simulink library "EngineSystemSubmodel"  (R2014b)
settings: Solver=ode45  StartTime=0.0  StopTime=10.0  FixedStep=1e-4  RelTol=1e-3
values from neighbouring files (symbols this model uses):
  D_turb_wheel = TC.TC_map.turb.D_wheel    [init_MVM.m]
  delta = 2    [Init8RTFLEX68D.m]    (also in Untitled2.m = fcn(p); fcn.m = zeros(size(p)))
  eta_turb_max = TC.TC_map.turb.eff_max    [init_MVM.m]
  flow_coeff_turb = [-1.585326540339;-4.823836967181;1.5853156139822]    [Init8RTFLEX68D.m]    (also in init_MVM.m = TC.TC_map.turb.flow_fit_coeff)
  fs = 0.0683    [Init8RTFLEX68D.m]    (also in NOxProcessGUI.m = varargin{2}; initHybrid.m; initMV.m; init_MVM.m = 0.0682925799315)
  genset = generators(1)    [runTempCyl4S.m]
  J_tc = TC.SAE_map_comp.inertia    [init_MVM.m]
  kai = 1.7    [Init8RTFLEX68D.m]
  Kb = 1*ones(engines,1)    [initHybrid.m]    (also in initMV.m; init_MVM.m = 1; init_ele.m = 1)
  Kd = 20*ones(engines,1)    [initHybrid.m]    (also in initMV.m; init_MVM.m = 10; init_ele.m = 20)
  Ki = 20*ones(engines,1)    [initHybrid.m]    (also in initMV.m; init_MVM.m = 10; init_ele.m = 20)
  Kp = 20*ones(engines,1)    [initHybrid.m]    (also in initMV.m; init_MVM.m = 10; init_ele.m = 20)
  Load_amp = x(4) + xRef(i)    [GetErrGensetResp.m]    (also in runsimulation.m = 0.55; runsimulationRecovery.m = InitialLoad(jj) + LoadStep(ii))
  Load_bias = x(4)    [GetErrGensetResp.m]    (also in runsimulation.m = 0.15; runsimulationRecovery.m = InitialLoad(jj))
  Load_index = 1    [GetErrGensetResp.m]    (also in runsimulation.m; runsimulationRecovery.m)
  N = x*noMol    [NOxProcessGUI.m]    (also in initHybrid.m = .1*ones(engines,1); initMV.m = .1*ones(engines,1); init_ele.m = 0.1)
  omegat0 = RPM_TC_initial/30*pi    [init_MVM.m]
  Start_time = 50    [GetErrGensetResp.m]    (also in runsimulation.m; runsimulationRecovery.m)
  T_load = 1    [GetErrGensetResp.m]    (also in runsimulation.m; runsimulationRecovery.m)
  T_ref_turb = TC.TC_map.turb.T_ref    [init_MVM.m]
  u0 = 0.2    [init_MVM.m]
  Uc_opt = TC.TC_map.turb.Uc_opt    [init_MVM.m]
  uMax = 1.5*ones(engines,1)    [initHybrid.m]    (also in initMV.m; init_MVM.m = 1.1; init_ele.m = 1.1)
  uMin = 0*ones(engines,1)    [initHybrid.m]    (also in initMV.m; init_MVM.m = 0.1; init_ele.m = 0.1)
undefined symbols (not defined in the file or in its folder): CAIPO, control, CV, cyl, eng, engSCont, omega0, rhoG0, Td, Ti, turbo, u_max, volDisp, vSCont, vSDes
undefined symbols (not defined in the file): comp_eff_map, comp_flow_map, n288_rep, npr, nsp, pr_rep, vComp
libraries: EngineSystemSubmodel x167, simulink x2
(part 4 of 5)

== system EngineSystemSubmodel/Components/TurbochargerFullModel ==
  pTFuComp : Inport
  pTFdComp : Inport  Port=2
  pTFuTurb : Inport  Port=3
  pTFdTurb : Inport  Port=4
  CompressorFullMap : EngineSystemSubmodel/Flow Restriction/CompressorFullMap  comp=turbo.comp
  Friction : Subsystem
  Gain : Gain  Gain=1/turbo.jTC
  Integrator : Integrator  InitialCondition=turbo.jTC*turbo.omegaT0
  Sum : Sum  Inputs=--+
  TurbineFullMap : EngineSystemSubmodel/Flow Restriction/TurbineFullMap  turb=turbo.turb
  dmEmbuComp : Outport
  dmEmbdComp : Outport  Port=2
  effComp : Outport  Port=3
  effComp1 : Outport  Port=4
  dmEmbuTurb : Outport  Port=5
  dmEmbdTurb : Outport  Port=6
  effTurb : Outport  Port=7
  TdTurb : Outport  Port=8
  wires:
  Integrator/1 -> Gain/1
  TurbineFullMap/3 -> Sum/3  "tqTurb"
  Sum/1 -> Integrator/1
  TurbineFullMap/4 -> effTurb/1  "etaTurb"
  Gain/1 -> TurbineFullMap/3, CompressorFullMap/3, Friction/1(In1)  "omegaTC"
  pTFdTurb/1 -> TurbineFullMap/2
  CompressorFullMap/3 -> Sum/2  "tqComp"
  TurbineFullMap/2 -> dmEmbdTurb/1
  pTFuComp/1 -> CompressorFullMap/1
  CompressorFullMap/1 -> dmEmbuComp/1
  pTFuTurb/1 -> TurbineFullMap/1
  CompressorFullMap/2 -> dmEmbdComp/1
  CompressorFullMap/4 -> effComp/1  "etaComp"
  pTFdComp/1 -> CompressorFullMap/2
  TurbineFullMap/1 -> dmEmbuTurb/1
  Friction/1(Out1) -> Sum/1  "tqFricTC"
  TurbineFullMap/5 -> TdTurb/1  "TAComp"
  CompressorFullMap/5 -> effComp1/1

== system EngineSystemSubmodel/Components/TurbochargerMV ==
  pTF_c_u : Inport
  pTF_c_d : Inport  Port=2
  pTF_t_u : Inport  Port=3
  pTF_t_d : Inport  Port=4
  Compressor : EngineSystemSubmodel/Flow Restriction/Compressor  comp=turbo.comp
  Gain : Gain  Gain=1/J_tc
  Integrator : Integrator  InitialCondition=omegat0*J_tc
  Sum : Sum  Inputs=-|+
  TurbineMV : EngineSystemSubmodel/Flow Restriction/TurbineMV  fs=fs  flow_coeff_turb=flow_coeff_turb  D_turb_wheel=D_turb_wheel  Uc_opt=Uc_opt  eta_turb_max=eta_turb_max
  dmEmb_c_u : Outport
  dmEmb_c_d : Outport  Port=2
  dmEmb_t_u : Outport  Port=3
  dmEmb_t_d : Outport  Port=4
  T_t_d_calc : Outport  Port=5
  eta_c : Outport  Port=6
  eta_t : Outport  Port=7
  wires:
  TurbineMV/5 -> eta_t/1
  TurbineMV/3 -> Sum/2  "Tqt"
  TurbineMV/1 -> dmEmb_t_u/1
  Compressor/1 -> dmEmb_c_u/1
  Gain/1 -> Compressor/3, TurbineMV/3  "omegat"
  Compressor/2 -> dmEmb_c_d/1
  Integrator/1 -> Gain/1
  Sum/1 -> Integrator/1
  Compressor/3 -> Sum/1  "Tqc"
  TurbineMV/2 -> dmEmb_t_d/1
  TurbineMV/4 -> T_t_d_calc/1
  pTF_c_d/1 -> Compressor/2
  pTF_c_u/1 -> Compressor/1
  pTF_t_u/1 -> TurbineMV/1
  pTF_t_d/1 -> TurbineMV/2
  Compressor/4 -> eta_c/1

== system EngineSystemSubmodel/Components/WasteGate ==
  pTF_u : Inport
  pTF_d : Inport  Port=2
  pTFScav : Inport  Port=3
  dmEmbExh : Inport  Port=4
  Demux : Demux  Outputs=3
  Demux1 : Demux  Outputs=3
  Demux2 : Demux  Outputs=3
  IdealNozzle : EngineSystemSubmodel/Flow Restriction/IdealNozzle
  S-Function : S-Function  FunctionName=lowPassFilterBW4  Parameters=BW,y0  EnableBusSupport=off  mask{BW=eng.control.WG.LPBWdmExhBypass, y0=0}
      mask prompts: BW "Bandwidth [Hz]"; y0 "Initial output"
  S-Function1 : S-Function  FunctionName=lowPassFilterBW4  Parameters=BW,y0  EnableBusSupport=off  mask{BW=eng.control.WG.LPBWdmExh, y0=0}
      mask prompts: BW "Bandwidth [Hz]"; y0 "Initial output"
  Terminator{,1..5} (6 alike) : Terminator
  wasteGateControl : Subsystem  mask{Kp=eng.control.WG.Kp, Ti=eng.control.WG.Ti, K_b=eng.control.WG.Kb, max=eng.control.WG.uMax, min=eng.control.WG.uMin, bypassRatio=eng.control.WG.Ratio, upper=eng.control.WG.upperOpenSPWG, lower=eng.control.WG.lowerCloseSPWG}
      mask prompts: Kp "Proportional gain"; Ti "Integral time constant"; K_b "Back calculation gain for anti-windup"; max "Maximum allowable valve opening"; min "Maximum allowable valve opening"; bypassRatio "Bypass ratio"; upper "Upper bound for opening waste gate"; lower "Lower bound for closing waste gate"
      mask TypeOptions Kp: Gain/Kp | Gain2/Kp
      mask TypeOptions Ti: Gain1/Ti
      mask TypeOptions K_b: Gain3/K_b
      mask TypeOptions max: Saturation/max
      mask TypeOptions min: Saturation/min
      mask TypeOptions bypassRatio: Constant1/bypassRatio
      mask TypeOptions upper: S-Function/upper
      mask TypeOptions lower: S-Function/lower
  dmEmb_u : Outport
  dmEmb_d : Outport  Port=2
  wires:
  Demux2/3 -> Terminator5/1
  Demux2/2 -> Terminator4/1
  Demux2/1 -> S-Function1/1
  dmEmbExh/1 -> Demux2/1
  Demux1/3 -> Terminator3/1
  Demux1/2 -> Terminator2/1
  Demux1/1 -> S-Function/1
  IdealNozzle/2 -> Demux1/1, dmEmb_d/1
  Demux/3 -> Terminator1/1
  Demux/2 -> Terminator/1
  Demux/1 -> wasteGateControl/3(pScav)
  S-Function/1 -> wasteGateControl/1(dmExhBypass)
  pTFScav/1 -> Demux/1
  S-Function1/1 -> wasteGateControl/2(dmExhTotal)
  pTF_d/1 -> IdealNozzle/3
  pTF_u/1 -> IdealNozzle/2
  wasteGateControl/1(wasteGateOpen) -> IdealNozzle/1, wasteGateControl/4(u saturated)
  IdealNozzle/1 -> dmEmb_u/1

== system EngineSystemSubmodel/Control System/ECSParamId ==
  Tq : Inport
  omegaE : Inport  Port=2
  RPMRef : Inport  Port=3
  dmf : Inport  Port=4
  pMax : Inport  Port=5
  pCyl : Inport  Port=6
  vCyl : Inport  Port=7
  exhVVOpen : Inport  Port=8
  dQCyl : Inport  Port=9
  BSFCRef : Inport  Port=10
  dQCylREf : Inport  Port=11
  Constant : Constant  Value=1e-6
  Constant1 : Constant  Value=exhVVStart  mask{exhVVStart=eng.control.EVO}
      mask prompts: exhVVStart "EVO timing (0.96~1.2)"
  Constant4 : Constant  Value=deltaPCombRef  mask{deltaPCombRef=control.inj.deltaPCombRef}
      mask prompts: deltaPCombRef "Reference pressure rise due to combustion"
  EVCControl : Subsystem  mask{Kp=control.EVC.Kp, Ti=control.EVC.Ti, max=control.EVC.uMax, min=control.EVC.uMin}
      mask prompts: Kp "Proportional gain"; Ti "Integral time constant"; max "Maximum allowable output"; min "Minimum allowable output"
  Gain : Gain  Gain=30/pi/eng.RPMMax
  Gain1 : Gain  Gain=1e-5
  Gain2 : Gain  Gain=3.6e9
  Gain3 : Gain  Gain=1e-5
  Gain4 : Gain  Gain=1/eng.RPMMax
  Gain5 : Gain  Gain=1/eng.nCyl
  InjectionControl : Subsystem  mask{Kp=control.inj.Kp, Ti=control.inj.Ti, max=control.inj.uMax, min=control.inj.uMin}
      mask prompts: Kp "Proportional gain"; Ti "Integral time constant"; max "Maximum allowable output"; min "Minimum allowable output"
  PIDControlAntiWinding : EngineSystemSubmodel/Control System/PIDControlAntiWinding  Kp=control.gov.Kp  Td=control.gov.Td  N=control.gov.N  Ti=control.gov.Ti  uMax=control.gov.uMax  uMin=control.gov.uMin  u0=control.gov.u0  Kb=control.gov.Kb
  Product : Product  Inputs=*/
  Product1 : Product
  Sum : Sum  Inputs=|++
  Sum1 : Sum  Inputs=|+-
  Sum2 : Sum  Inputs=|-+
  dQCylLPFilterBW1 : S-Function  FunctionName=lowPassFilterBW4  Parameters=BW,y0  EnableBusSupport=off  mask{BW=eng.control.HRejId.LPBWQCyl, y0=0}
      mask prompts: BW "Bandwidth [Hz]"; y0 "Initial output"
  dmfLPFilterBW4 : S-Function  FunctionName=lowPassFilterBW4  Parameters=BW,y0  EnableBusSupport=off  mask{BW=eng.control.pMax.LPBWdmf, y0=eng.BSFC0*(eng.engLoad0*eng.Pe)/3.6e9}
      mask prompts: BW "Bandwidth [Hz]"; y0 "Initial output"
  engSpeedLPFilterBW1 : S-Function  FunctionName=lowPassFilterBW4  Parameters=BW,y0  EnableBusSupport=off  mask{BW=100, y0=0}
      mask prompts: BW "Bandwidth [Hz]"; y0 "Initial output"
  engSpeedLPFilterBW4 : S-Function  FunctionName=lowPassFilterBW4  Parameters=BW,y0  EnableBusSupport=off  mask{BW=eng.control.gov.LPBW, y0=eng.omegaE0}
      mask prompts: BW "Bandwidth [Hz]"; y0 "Initial output"
  maxPCylMaxControl : Subsystem  mask{Kp=control.pMax.Kp, Ti=control.pMax.Ti, max=control.pMax.uMax, min=control.pMax.uMin}
      mask prompts: Kp "Proportional gain"; Ti "Integral time constant"; max "Maximum allowable output"; min "Minimum allowable output"
  pCompCalc : EngineSystemSubmodel/EngineOperatingParameterCalculation/pCompCalc  vComp=eng.cyl(1).dim.vComp
  powLPFilterBW4 : S-Function  FunctionName=lowPassFilterBW4  Parameters=BW,y0  EnableBusSupport=off  mask{BW=eng.control.pMax.LPBWPow, y0=eng.engLoad0*eng.Pe}
      mask prompts: BW "Bandwidth [Hz]"; y0 "Initial output"
  tempWallControl : Subsystem  mask{Kp=control.HRejId.Kp, Ti=control.HRejId.Ti, swTWCont=control.HRejId.sw}
      mask prompts: Kp "Proportional gain"; Ti "Integral time constant"; swTWCont "Switch ON/OFF for TWall identification"
  uGov : Outport
  phiInj : Outport  Port=2
  cAStartNom : Outport  Port=3
  dCALiftUp : Outport  Port=4
  TWall : Outport  Port=5
  wires:
  Gain5/1 -> tempWallControl/2(dQCylRef)  "dQCyl1Ref"
  Gain4/1 -> PIDControlAntiWinding/2  "engSpeedRefPU"
  Gain/1 -> PIDControlAntiWinding/1  "engSpeedPU"
  Gain1/1 -> EVCControl/1(pComp)  "pCompBar"
  engSpeedLPFilterBW1/1 -> Gain1/1, Sum1/2  "pComp"
  BSFCRef/1 -> maxPCylMaxControl/2(BSFCRef)  "BSFCREf"
  omegaE/1 -> Product1/1, engSpeedLPFilterBW4/1
  engSpeedLPFilterBW4/1 -> Gain/1  "omegaELP"
  RPMRef/1 -> Gain4/1
  PIDControlAntiWinding/1 -> PIDControlAntiWinding/3, uGov/1  "uGov"
  Product1/1 -> powLPFilterBW4/1  "powInst"
  Constant1/1 -> cAStartNom/1  "CAStartNom"
  powLPFilterBW4/1 -> Sum/2  "powLP"
  dmf/1 -> dmfLPFilterBW4/1
  Sum/1 -> Product/2
  Product/1 -> Gain2/1
  Gain2/1 -> maxPCylMaxControl/1(BSFCMeas)  "BSFC"
  pCyl/1 -> pCompCalc/1
  vCyl/1 -> pCompCalc/2
  tempWallControl/1(TWall) -> pCompCalc/3, TWall/1  "tempWall"
  pMax/1 -> Sum1/1
  Sum1/1 -> Gain3/1  "deltaPComb"
  Gain3/1 -> InjectionControl/1(deltaPComb), Sum2/1
  maxPCylMaxControl/1(pMaxRef) -> Sum2/2  "pMaxRef"
  Sum2/1 -> EVCControl/2(pCompRef)  "pCompRef"
  Constant4/1 -> InjectionControl/2(deltaPCombRef)
  Tq/1 -> Product1/2
  dmfLPFilterBW4/1 -> Product/1  "dmfLP"
  Constant/1 -> Sum/1
  exhVVOpen/1 -> pCompCalc/4
  pCompCalc/1 -> engSpeedLPFilterBW1/1
  InjectionControl/1(phiInjRef) -> phiInj/1  "phiInj"
  EVCControl/1(EVCRef) -> dCALiftUp/1  "EVC"
  dQCyl/1 -> dQCylLPFilterBW1/1
  dQCylLPFilterBW1/1 -> tempWallControl/1(dQCyl)  "dQCyl1"
  dQCylREf/1 -> Gain5/1

== system EngineSystemSubmodel/Control System/ECSTrans ==
  Tq : Inport
  omegaE : Inport  Port=2
  RPMRef : Inport  Port=3
  dmf : Inport  Port=4
  dme : Inport  Port=5
  Constant : Constant  Value=1e-6
  Constant1 : Constant  Value=exhVVStart  mask{exhVVStart=control.EVO}
      mask prompts: exhVVStart "EVO timing (0.96~1.2)"
  Gain : Gain  Gain=30/pi/eng.RPMMax
  Gain1 : Gain  Gain=1/eng.Pe
  Gain2 : Gain  Gain=3.6e9
  Gain3 : Gain  Gain=3.6e6
  Gain4 : Gain  Gain=1/eng.RPMMax
  PIDControlAntiWinding : EngineSystemSubmodel/Control System/PIDControlAntiWinding  Kp=control.gov.Kp  Td=control.gov.Td  N=control.gov.N  Ti=control.gov.Ti  uMax=control.gov.uMax  uMin=control.gov.uMin  u0=control.gov.u0  Kb=control.gov.Kb
  Product : Product  Inputs=*/
  Product1 : Product
  Product2 : Product  Inputs=*/
  S-Function : S-Function  FunctionName=interpolateDescend  Parameters=xREf,yRef  EnableBusSupport=off  mask{xREf=eng.control.inj.phiInjxRef, yRef=eng.control.inj.phiInjyRef}
      mask prompts: xREf "x Reference array to interpolate"; yRef "y Reference array to interpolate"
  S-Function1 : S-Function  FunctionName=interpolateDescend  Parameters=xREf,yRef  EnableBusSupport=off  mask{xREf=eng.control.EVC.EVCxRef, yRef=eng.control.EVC.EVCyRef}
      mask prompts: xREf "x Reference array to interpolate"; yRef "y Reference array to interpolate"
  S-Function2 : S-Function  FunctionName=lowPassFilterBW4  Parameters=BW,y0  EnableBusSupport=off  mask{BW=eng.control.dmfLP.BW, y0=eng.BSFC0*(eng.engLoad0*eng.Pe)/3.6e9}
      mask prompts: BW "Bandwidth [Hz]"; y0 "Initial output"
  S-Function3 : S-Function  FunctionName=lowPassFilterBW4  Parameters=BW,y0  EnableBusSupport=off  mask{BW=eng.control.powLP.BW, y0=eng.control.powLP.pow0}
      mask prompts: BW "Bandwidth [Hz]"; y0 "Initial output"
  S-Function4 : S-Function  FunctionName=lowPassFilterBW4  Parameters=BW,y0  EnableBusSupport=off  mask{BW=eng.control.gov.LPBW, y0=eng.omegaE0}
      mask prompts: BW "Bandwidth [Hz]"; y0 "Initial output"
  S-Function5 : S-Function  FunctionName=lowPassFilterBW4  Parameters=BW,y0  EnableBusSupport=off  mask{BW=eng.control.dmeLP.BW, y0=eng.control.dmeLP.dme0}
      mask prompts: BW "Bandwidth [Hz]"; y0 "Initial output"
  Sum : Sum  Inputs=|++
  Terminator1 : Terminator
  Terminator2 : Terminator
  uGov : Outport
  phiInj : Outport  Port=2
  cAStartNom : Outport  Port=3
  dCALiftUp : Outport  Port=4
  wires:
  Gain3/1 -> Terminator1/1  "BSEF"
  Product2/1 -> Gain3/1
  S-Function5/1 -> Product2/1  "dmeLP"
  dme/1 -> S-Function5/1
  omegaE/1 -> Product1/1, S-Function4/1
  S-Function4/1 -> Gain/1  "omegaELP"
  Gain/1 -> PIDControlAntiWinding/1  "engSpeedPU"
  RPMRef/1 -> Gain4/1
  PIDControlAntiWinding/1 -> PIDControlAntiWinding/3, uGov/1  "uGov"
  Product1/1 -> S-Function3/1  "powInst"
  Constant1/1 -> cAStartNom/1
  S-Function3/1 -> Product2/2, Sum/2, Gain1/1  "powLP"
  Gain1/1 -> S-Function1/1, S-Function/1  "PL"
  dmf/1 -> S-Function2/1
  Sum/1 -> Product/2
  Product/1 -> Gain2/1
  Gain2/1 -> Terminator2/1  "BSFC"
  Gain4/1 -> PIDControlAntiWinding/2  "engSpeedRefPU"
  Tq/1 -> Product1/2
  S-Function2/1 -> Product/1  "dmfLP"
  Constant/1 -> Sum/1
  S-Function/1 -> phiInj/1
  S-Function1/1 -> dCALiftUp/1

== system EngineSystemSubmodel/Control System/ECSTrans1 ==
  Tq : Inport
  omegaE : Inport  Port=2
  RPMRef : Inport  Port=3
  dmf : Inport  Port=4
  dme : Inport  Port=5
  vS : Inport  Port=6
  vSRef : Inport  Port=7
  Constant : Constant  Value=1e-6
  Constant1 : Constant  Value=exhVVStart  mask{exhVVStart=eng.control.EVO}
      mask prompts: exhVVStart "EVO timing (0.96~1.2)"
  Gain : Gain  Gain=30/pi/eng.RPMMax
  Gain1 : Gain  Gain=1/eng.Pe
  Gain11 : Gain  Gain=vSCont
  Gain12 : Gain  Gain=engSCont
  Gain2 : Gain  Gain=3.6e9
  Gain3 : Gain  Gain=3.6e6
  Gain4 : Gain  Gain=1/eng.RPMMax
  Gain8 : Gain  Gain=1/vSDes
  Integrator : Integrator
  PIDControlAntiWinding : EngineSystemSubmodel/Control System/PIDControlAntiWinding  Kp=control.gov.Kp  Td=control.gov.Td  N=control.gov.N  Ti=control.gov.Ti  uMax=control.gov.uMax  uMin=control.gov.uMin  u0=control.gov.u0  Kb=control.gov.Kb
  PIDControlAntiWinding1 : EngineSystemSubmodel/Control System/PIDControlAntiWinding  Kp=control.speed.Kp  Td=control.speed.Td  N=control.speed.N  Ti=control.speed.Ti  uMax=control.speed.uMax  uMin=control.speed.uMin  u0=control.speed.u0  Kb=control.speed.Kb
  Product : Product  Inputs=*/
  Product1 : Product
  Product2 : Product  Inputs=*/
  S-Function : S-Function  FunctionName=interpolateDescend  Parameters=xREf,yRef  EnableBusSupport=off  mask{xREf=eng.control.inj.phiInjxRef, yRef=eng.control.inj.phiInjyRef}
      mask prompts: xREf "x Reference array to interpolate"; yRef "y Reference array to interpolate"
  S-Function1 : S-Function  FunctionName=interpolateDescend  Parameters=xREf,yRef  EnableBusSupport=off  mask{xREf=eng.control.EVC.EVCxRef, yRef=eng.control.EVC.EVCyRef}
      mask prompts: xREf "x Reference array to interpolate"; yRef "y Reference array to interpolate"
  S-Function2 : S-Function  FunctionName=lowPassFilterBW4  Parameters=BW,y0  EnableBusSupport=off  mask{BW=eng.control.dmfLP.BW, y0=eng.BSFC0*(eng.engLoad0*eng.Pe)/3.6e9}
      mask prompts: BW "Bandwidth [Hz]"; y0 "Initial output"
  S-Function3 : S-Function  FunctionName=lowPassFilterBW4  Parameters=BW,y0  EnableBusSupport=off  mask{BW=eng.control.powLP.BW, y0=eng.control.powLP.pow0}
      mask prompts: BW "Bandwidth [Hz]"; y0 "Initial output"
  S-Function4 : S-Function  FunctionName=lowPassFilterBW4  Parameters=BW,y0  EnableBusSupport=off  mask{BW=eng.control.gov.LPBW, y0=eng.omegaE0}
      mask prompts: BW "Bandwidth [Hz]"; y0 "Initial output"
  S-Function5 : S-Function  FunctionName=lowPassFilterBW4  Parameters=BW,y0  EnableBusSupport=off  mask{BW=eng.control.dmeLP.BW, y0=eng.control.dmeLP.dme0}
      mask prompts: BW "Bandwidth [Hz]"; y0 "Initial output"
  S-Function6 : EngineSystemSubmodel/Control System/ECSTrans1/S-Function4  BW=eng.control.speed.LPBW  y0=vS0
  Sum : Sum  Inputs=|++
  Sum2 : Sum  Inputs=|++
  Terminator : Terminator
  Terminator1 : Terminator
  Terminator2 : Terminator
  uGov : Outport
  phiInj : Outport  Port=2
  cAStartNom : Outport  Port=3
  dCALiftUp : Outport  Port=4
  wires:
  S-Function1/1 -> dCALiftUp/1
  S-Function/1 -> phiInj/1
  Constant/1 -> Sum/1
  S-Function2/1 -> Product/1  "dmfLP"
  Tq/1 -> Product1/2
  Gain4/1 -> PIDControlAntiWinding/2  "engSpeedRefPU"
  Gain2/1 -> Terminator2/1  "BSFC"
  Product/1 -> Gain2/1
  Sum/1 -> Product/2
  dmf/1 -> S-Function2/1
  Gain1/1 -> S-Function/1, S-Function1/1  "PL"
  S-Function3/1 -> Gain1/1, Sum/2, Product2/2  "powLP"
  Constant1/1 -> cAStartNom/1
  Product1/1 -> Integrator/1, S-Function3/1  "powInst"
  RPMRef/1 -> Gain4/1
  Gain/1 -> PIDControlAntiWinding/1  "engSpeedPU"
  S-Function4/1 -> Gain/1  "omegaELP"
  omegaE/1 -> S-Function4/1, Product1/1
  dme/1 -> S-Function5/1
  S-Function5/1 -> Product2/1  "dmeLP"
  Product2/1 -> Gain3/1
  Gain3/1 -> Terminator1/1  "BSEF"
  Integrator/1 -> Terminator/1  "workShaft"
  Sum2/1 -> uGov/1
  Gain12/1 -> Sum2/2
  Gain11/1 -> Sum2/1
  PIDControlAntiWinding1/1 -> PIDControlAntiWinding1/3, Gain11/1
  Gain8/1 -> PIDControlAntiWinding1/1
  S-Function6/1 -> Gain8/1
  vS/1 -> S-Function6/1
  vSRef/1 -> PIDControlAntiWinding1/2
  PIDControlAntiWinding/1 -> PIDControlAntiWinding/3, Gain12/1

== system EngineSystemSubmodel/Control System/ECSTransSmokeLim ==
  Tq : Inport
  omegaE : Inport  Port=2
  RPMRef : Inport  Port=3
  dmf : Inport  Port=4
  dme : Inport  Port=5
  vS : Inport  Port=6
  vSRef : Inport  Port=7
  pTFVAR : Inport  Port=8
  volEff : Inport  Port=9
  Bus Selector : BusSelector  OutputSignals=p,T
  Compare To Constant : simulink/Logic and Bit Operations/Compare To Constant  relop=<=  const=(eng.RPMMax/30*pi)*0.1  OutDataTypeStr=boolean
  Constant : Constant  Value=1e-6
  Constant1 : Constant  Value=exhVVStart  mask{exhVVStart=eng.control.EVO}
      mask prompts: exhVVStart "EVO timing (0.96~1.2)"
  Gain : Gain  Gain=30/pi/eng.RPMMax
  Gain1 : Gain  Gain=1/eng.Pe
  Gain11 : Gain  Gain=vSCont
  Gain12 : Gain  Gain=engSCont
  Gain2 : Gain  Gain=3.6e9
  Gain3 : Gain  Gain=3.6e6
  Gain4 : Gain  Gain=1/eng.RPMMax
  Gain5 : Gain  Gain=vSCont
  Gain6 : Gain  Gain=engSCont
  Gain8 : Gain  Gain=1/vSDes
  Integrator : Integrator
  PIDControlAntiWinding : EngineSystemSubmodel/Control System/PIDControlAntiWinding  Kp=control.gov.Kp  Td=control.gov.Td  N=control.gov.N  Ti=control.gov.Ti  uMax=control.gov.uMax  uMin=control.gov.uMin  u0=control.gov.u0  Kb=control.gov.Kb
  PIDControlAntiWinding1 : EngineSystemSubmodel/Control System/PIDControlAntiWinding  Kp=control.speed.Kp  Td=control.speed.Td  N=control.speed.N  Ti=control.speed.Ti  uMax=control.speed.uMax  uMin=control.speed.uMin  u0=control.speed.u0  Kb=control.speed.Kb
  Product : Product  Inputs=*/
  Product1 : Product
  Product2 : Product  Inputs=*/
  S-Function : S-Function  FunctionName=interpolateDescend  Parameters=xREf,yRef  EnableBusSupport=off  mask{xREf=eng.control.inj.phiInjxRef, yRef=eng.control.inj.phiInjyRef}
      mask prompts: xREf "x Reference array to interpolate"; yRef "y Reference array to interpolate"
  S-Function1 : S-Function  FunctionName=interpolateDescend  Parameters=xREf,yRef  EnableBusSupport=off  mask{xREf=eng.control.EVC.EVCxRef, yRef=eng.control.EVC.EVCyRef}
      mask prompts: xREf "x Reference array to interpolate"; yRef "y Reference array to interpolate"
  S-Function2 : S-Function  FunctionName=lowPassFilterBW4  Parameters=BW,y0  EnableBusSupport=off  mask{BW=eng.control.dmfLP.BW, y0=eng.BSFC0*(eng.engLoad0*eng.Pe)/3.6e9}
      mask prompts: BW "Bandwidth [Hz]"; y0 "Initial output"
  S-Function3 : S-Function  FunctionName=lowPassFilterBW4  Parameters=BW,y0  EnableBusSupport=off  mask{BW=eng.control.powLP.BW, y0=eng.control.powLP.pow0}
      mask prompts: BW "Bandwidth [Hz]"; y0 "Initial output"
  S-Function4 : S-Function  FunctionName=lowPassFilterBW4  Parameters=BW,y0  EnableBusSupport=off  mask{BW=eng.control.gov.LPBW, y0=eng.omegaE0}
      mask prompts: BW "Bandwidth [Hz]"; y0 "Initial output"
  S-Function5 : S-Function  FunctionName=lowPassFilterBW4  Parameters=BW,y0  EnableBusSupport=off  mask{BW=eng.control.dmeLP.BW, y0=eng.control.dmeLP.dme0}
      mask prompts: BW "Bandwidth [Hz]"; y0 "Initial output"
  S-Function6 : EngineSystemSubmodel/Control System/ECSTrans1/S-Function4  BW=eng.control.speed.LPBW  y0=vS0
  Smoke Limiter : EngineSystemSubmodel/Control System/Smoke Limiter
  Stop Simulation : Stop
  Sum : Sum  Inputs=|++
  Sum2 : Sum  Inputs=|++
  Terminator{,1..3} (4 alike) : Terminator
  uGov : Outport
  phiInj : Outport  Port=2
  cAStartNom : Outport  Port=3
  dCALiftUp : Outport  Port=4
  wires:
  Compare To Constant/1 -> Stop Simulation/1
  PIDControlAntiWinding/1 -> Gain12/1
  vSRef/1 -> PIDControlAntiWinding1/2
  vS/1 -> S-Function6/1
  S-Function6/1 -> Gain8/1
  Gain8/1 -> PIDControlAntiWinding1/1
  PIDControlAntiWinding1/1 -> Gain11/1
  Gain11/1 -> Sum2/1
  Gain12/1 -> Sum2/2
  Sum2/1 -> Smoke Limiter/1
  Integrator/1 -> Terminator/1  "workShaft"
  Gain3/1 -> Terminator1/1  "BSEF"
  Product2/1 -> Gain3/1
  S-Function5/1 -> Product2/1  "dmeLP"
  dme/1 -> S-Function5/1
  omegaE/1 -> Product1/1, S-Function4/1, Compare To Constant/1
  S-Function4/1 -> Gain/1  "omegaELP"
  Gain/1 -> PIDControlAntiWinding/1  "engSpeedPU"
  RPMRef/1 -> Gain4/1
  Product1/1 -> S-Function3/1, Integrator/1  "powInst"
  Constant1/1 -> cAStartNom/1
  S-Function3/1 -> Product2/2, Sum/2, Gain1/1  "powLP"
  Gain1/1 -> S-Function1/1, S-Function/1  "PL"
  dmf/1 -> S-Function2/1
  Sum/1 -> Product/2
  Product/1 -> Gain2/1
  Gain2/1 -> Terminator2/1  "BSFC"
  Gain4/1 -> PIDControlAntiWinding/2  "engSpeedRefPU"
  Tq/1 -> Product1/2
  S-Function2/1 -> Product/1  "dmfLP"
  Constant/1 -> Sum/1
  S-Function/1 -> phiInj/1
  S-Function1/1 -> dCALiftUp/1
  Smoke Limiter/1 -> Gain5/1, Gain6/1, uGov/1  "uGov"
  volEff/1 -> Smoke Limiter/4
  pTFVAR/1 -> Bus Selector/1
  Bus Selector/2 -> Smoke Limiter/3  "<T>"
  Bus Selector/1 -> Smoke Limiter/2  "<p>"
  Gain5/1 -> PIDControlAntiWinding1/3
  Gain6/1 -> PIDControlAntiWinding/3
  Smoke Limiter/2 -> Terminator3/1  "uMax"

== system EngineSystemSubmodel/Control System/Governor ==
  u saturated : Inport
  omega_pu : Inport  Port=2
  "wNL, pu" : Inport  Port=3
  "pe, pu" : Inport  Port=4
  Constant : Constant
  Gain : Gain  Gain=genset.governor.droop
  PID controller : Subsystem
  Product : Product  RndMeth=Zero
  Sum : Sum  Inputs=|+-
  Sum1 : Sum  Inputs=|+-
  u : Outport
  wires:
  omega_pu/1 -> PID controller/2(omega_pu), Sum/2
  "pe, pu"/1 -> Gain/1
  u saturated/1 -> PID controller/3(u saturated)
  Sum1/1 -> Product/2
  Constant/1 -> Sum1/1
  "wNL, pu"/1 -> Product/1
  Product/1 -> Sum/1
  Sum/1 -> PID controller/1(e)
  Gain/1 -> Sum1/2
  PID controller/1(u) -> u/1  "u"

== system EngineSystemSubmodel/Control System/Governor_SpeedControl ==
  u saturated : Inport
  omega_pu : Inport  Port=2
  omega_pu_ref : Inport  Port=3
  PID controller : Subsystem  mask{Kp=Kp, Kd=Kd, N=N, Ki=Ki, Kb=Kb, omega0=omega0, u_max=u_max, u_min=u_min, u0=u0}
      mask prompts: Kp "Proportional gain"; Kd "Differtial gain"; N "Dirty derivative gain"; Ki "Integral gain"; Kb "Back-calculation gain"; omega0 "Initial speed"; u_max "Maximum output"; u_min "Minimum output"; u0 "Initial output"
  Sum : Sum  Inputs=|+-
  u : Outport
  wires:
  omega_pu/1 -> PID controller/2(omega_pu), Sum/2
  u saturated/1 -> PID controller/3(u saturated)
  omega_pu_ref/1 -> Sum/1
  Sum/1 -> PID controller/1(e)  "error"
  PID controller/1(u) -> u/1

== system EngineSystemSubmodel/Control System/PIDControlAntiWinding ==
  MV : Inport
  SP : Inport  Port=2
  uSat : Inport  Port=3
  S-Function : S-Function  FunctionName=SpeedController  Parameters=Kp,Td,N,Ti,Kb,uMax,uMin,u0  EnableBusSupport=off
  output : Outport
  wires:
  S-Function/1 -> output/1
  uSat/1 -> S-Function/3
  SP/1 -> S-Function/2
  MV/1 -> S-Function/1

== system EngineSystemSubmodel/Control System/Smoke Limiter ==
  u_gov : Inport
  p_air_manifold : Inport  Port=2
  T_air_manifold : Inport  Port=3
  vol_eff : Inport  Port=4
  Disp. Vol : Gain  Gain=eng.cyl(1).dim.vDisp
  Divide : Product  Inputs=/*
  Gain : Gain  Gain=eng.fs
  Gain1 : Gain  Gain=eng.control.smokeLim.FMax
  Gain2 : Gain  Gain=1/eng.cyl(1).comb.mqfCycMax
  LPFilterBW1 : EngineSystemSubmodel/Control System/LPFilterBW4  BW=eng.control.smokeLim.LPBW  y0=eng.scavRec.p0
  LPFilterBW4 : EngineSystemSubmodel/Control System/LPFilterBW4  BW=eng.control.smokeLim.LPBW  y0=eng.scavRec.T0
  LP_T0_2 : Subsystem
  MinMax : MinMax  Inputs=2
  Product : Product
  R_air : Gain  Gain=287
  u : Outport
  u_max : Outport  Port=2
  wires:
  LP_T0_2/1(Out1) -> Product/2
  LPFilterBW1/1 -> Divide/2
  LPFilterBW4/1 -> R_air/1
  Divide/1 -> Disp. Vol/1  "rho_air"
  p_air_manifold/1 -> LPFilterBW1/1
  R_air/1 -> Divide/1
  T_air_manifold/1 -> LPFilterBW4/1
  Disp. Vol/1 -> Product/1  "m_air_ideal"
  MinMax/1 -> u/1  "u"
  vol_eff/1 -> LP_T0_2/1(In1)  "eta_vol"
  Product/1 -> Gain/1  "m_a_cyl"
  u_gov/1 -> MinMax/1
  Gain/1 -> Gain1/1  "m_f_st"
  Gain1/1 -> Gain2/1  "m_f_max"
  Gain2/1 -> u_max/1, MinMax/2  "u_max"

== system EngineSystemSubmodel/Control System/Smoke Limiter MV ==
  u_gov : Inport
  p_air_manifold : Inport  Port=2
  T_air_manifold : Inport  Port=3
  vol_eff : Inport  Port=4
  Disp. Vol : Gain  Gain=Vd
  Divide : Product  Inputs=/*
  Gain : Gain  Gain=fs
  Gain1 : Gain  Gain=F_max
  Gain2 : Gain  Gain=1/m_f_cyc_max
  LP_T0_01 : Subsystem
  LP_T0_1 : Subsystem
  LP_T0_2 : Subsystem
  MinMax : MinMax  Inputs=2
  Product : Product
  R_air : Gain  Gain=287
  u : Outport
  u_max : Outport  Port=2
  wires:
  LP_T0_2/1(Out1) -> Product/2
  LP_T0_1/1(Out1) -> Divide/2
  LP_T0_01/1(Out1) -> R_air/1
  Divide/1 -> Disp. Vol/1  "rho_air"
  p_air_manifold/1 -> LP_T0_1/1(In1)
  R_air/1 -> Divide/1
  T_air_manifold/1 -> LP_T0_01/1(In1)
  Disp. Vol/1 -> Product/1  "m_air_ideal"
  MinMax/1 -> u/1  "u"
  vol_eff/1 -> LP_T0_2/1(In1)  "eta_vol"
  Product/1 -> Gain/1  "m_a_cyl"
  u_gov/1 -> MinMax/1
  Gain/1 -> Gain1/1  "m_f_st"
  Gain1/1 -> Gain2/1  "m_f_max"
  Gain2/1 -> u_max/1, MinMax/2  "u_max"

== system EngineSystemSubmodel/Control System/SpeedController ==
  MV : Inport
  SP : Inport  Port=2
  Demux : Demux  Outputs=[1 ]
  Mux : Mux  Inputs=[1 1 ]
  S-Function : S-Function  FunctionName=SpeedController  Parameters=Kp,Td,N,Ti,min,max,u0  EnableBusSupport=off
  output : Outport
  wires:
  MV/1 -> Mux/1
  SP/1 -> Mux/2
  Demux/1 -> output/1
  Mux/1 -> S-Function/1
  S-Function/1 -> Demux/1

== system EngineSystemSubmodel/Control Volume/ThdynCV2ZoneBG_VarVolBus ==
  dm : Inport
  dHCyl : Inport  Port=2
  dmb : Inport  Port=3
  dV : Inport  Port=4
  dmfb : Inport  Port=5
  dQCyl : Inport  Port=6
  FComb : Inport  Port=7
  phi : Inport  Port=8
  combState : Inport  Port=9
  dWCyl : Inport  Port=10
  Bus Creator : BusCreator
  Bus Creator1 : BusCreator
  S-Function : S-Function  FunctionName=ThdynCVNV2Zone  Parameters=eng.fs,cyl.comb.DPhiMix,cyl.comb.phiMix0,cyl.comb.alpha,eng.hn,CV.m0,CV.E0,CV.mb0,CV.V0,eng.nStroke  EnableBusSupport=off
  pTFVu : Outport
  pTFVb : Outport  Port=2
  wires:
  S-Function/8 -> Bus Creator1/1  "pb"
  dWCyl/1 -> S-Function/7
  FComb/1 -> S-Function/8
  combState/1 -> S-Function/10
  phi/1 -> S-Function/9
  dm/1 -> S-Function/1
  dmb/1 -> S-Function/2
  dV/1 -> S-Function/3
  dmfb/1 -> S-Function/4  "dmfb"
  dQCyl/1 -> S-Function/5
  dHCyl/1 -> S-Function/6
  Bus Creator/1 -> pTFVu/1
  S-Function/4 -> Bus Creator/4  "V"
  S-Function/3 -> Bus Creator/3  "F"
  S-Function/2 -> Bus Creator/2  "T"
  S-Function/1 -> Bus Creator/1  "p"
  S-Function/5 -> Bus Creator1/2  "Tb"
  S-Function/6 -> Bus Creator1/3  "F"
  S-Function/7 -> Bus Creator1/4  "Vb"
  Bus Creator1/1 -> pTFVb/1

== system EngineSystemSubmodel/Control Volume/ThdynCV2ZoneConv_VarVolBus ==
  dm : Inport
  dE : Inport  Port=2
  dmb : Inport  Port=3
  dV : Inport  Port=4
  dmfb : Inport  Port=5
  FComb : Inport  Port=6
  dQCyl : Inport  Port=7
  omega : Inport  Port=8
  phi : Inport  Port=9
  combState : Inport  Port=10
  mqf0 : Inport  Port=11
  Bus Creator : BusCreator
  Bus Creator1 : BusCreator
  Mux : Mux  Inputs=3
  S-Function : S-Function  FunctionName=ThdynCV2ZoneConv  Parameters=eng.fs,cyl.comb.DPhiMix,cyl.comb.phiMix0,cyl.comb.alpha,eng.hn,CV.p0,CV.T0,CV.F0,CV.V0,eng.nStroke  EnableBusSupport=off
  pTFVu : Outport
  pTFVb : Outport  Port=2
  wires:
  Bus Creator/1 -> pTFVu/1
  S-Function/4 -> Bus Creator/4  "V"
  S-Function/3 -> Bus Creator/3  "F"
  S-Function/2 -> Bus Creator/2  "T"
  S-Function/1 -> Bus Creator1/1, Bus Creator/1  "p"
  dm/1 -> Mux/1
  dE/1 -> Mux/2
  dmb/1 -> Mux/3
  Mux/1 -> S-Function/1
  dV/1 -> S-Function/2
  dmfb/1 -> S-Function/3  "dmfb"
  FComb/1 -> S-Function/4
  dQCyl/1 -> S-Function/5
  omega/1 -> S-Function/6
  phi/1 -> S-Function/7
  combState/1 -> S-Function/8
  mqf0/1 -> S-Function/9  "mqf"
  S-Function/5 -> Bus Creator1/2  "T"
  S-Function/6 -> Bus Creator1/3  "F"
  S-Function/7 -> Bus Creator1/4  "Vb"
  Bus Creator1/1 -> pTFVb/1

== system EngineSystemSubmodel/Control Volume/ThdynCVConv_VarVol ==
  dmEmb : Inport
  dV : Inport  Port=2
  Demux : Demux  Outputs=3
  Mux : Mux  Inputs=3
  S-Function : S-Function  FunctionName=ThdynCVConv  Parameters=eng.fs,CV.p0,CV.T0,CV.F0,CV.V0  EnableBusSupport=off
  pTF : Outport
  p : Outport  Port=2
  V : Outport  Port=3
  wires:
  Demux/1 -> S-Function/1
  Demux/2 -> S-Function/2
  Demux/3 -> S-Function/3
  dmEmb/1 -> Demux/1
  dV/1 -> S-Function/4
  S-Function/2 -> Mux/2
  S-Function/3 -> Mux/3
  S-Function/4 -> V/1
  Mux/1 -> pTF/1
  S-Function/1 -> p/1, Mux/1

== system EngineSystemSubmodel/Control Volume/ThdynCVConv_VarVolBus ==
  dm : Inport
  dE : Inport  Port=2
  dmb : Inport  Port=3
  dV : Inport  Port=4
  Bus Creator : BusCreator
  S-Function : S-Function  FunctionName=ThdynCVConv  Parameters=eng.fs,CV.p0,CV.T0,CV.F0,CV.V0  EnableBusSupport=off
  pTFV : Outport
  wires:
  dm/1 -> S-Function/1
  dE/1 -> S-Function/2
  dmb/1 -> S-Function/3
  dV/1 -> S-Function/4
  S-Function/1 -> Bus Creator/1  "p"
  S-Function/2 -> Bus Creator/2  "T"
  S-Function/3 -> Bus Creator/3  "F"
  S-Function/4 -> Bus Creator/4  "V"
  Bus Creator/1 -> pTFV/1

== system EngineSystemSubmodel/Control Volume/ThdynCV_FixVol ==
  dmEmb : Inport
  Constant_V : Constant  Value=CV.V0
  Demux : Demux  Outputs=3
  Integrator_E : Integrator  InitialCondition=CV.E0
  Integrator_m : Integrator  InitialCondition=CV.m0
  Integrator_mb : Integrator  InitialCondition=CV.mb0
  Mux : Mux  Inputs=3
  S-Function : S-Function  FunctionName=ThdynCV  Parameters=eng.fs  SFunctionModules=GetThdynCombGasZach.c GetPTF.c  EnableBusSupport=off
  pTF : Outport
  wires:
  Demux/1 -> Integrator_m/1
  dmEmb/1 -> Demux/1
  Demux/2 -> Integrator_E/1
  Demux/3 -> Integrator_mb/1
  Integrator_m/1 -> S-Function/1
  Integrator_E/1 -> S-Function/2
  Integrator_mb/1 -> S-Function/3
  Constant_V/1 -> S-Function/4
  S-Function/3 -> Mux/3
  S-Function/1 -> Mux/1
  Mux/1 -> pTF/1
  S-Function/2 -> Mux/2

== system EngineSystemSubmodel/Control Volume/ThdynCV_VarVol ==
  dmEmb : Inport
  dV : Inport  Port=2
  Demux : Demux  Outputs=3
  Integrator_E : Integrator  InitialCondition=CV.E0
  Integrator_V : Integrator  InitialCondition=CV.V0
  Integrator_m : Integrator  InitialCondition=CV.m0
  Integrator_mb : Integrator  InitialCondition=CV.mb0
  Mux : Mux  Inputs=3
  S-Function : S-Function  FunctionName=ThdynCV  Parameters=eng.fs  SFunctionModules=GetThdynCombGasZach.c GetPTF.c  EnableBusSupport=off
  pTF : Outport
  p : Outport  Port=2
  v : Outport  Port=3
  wires:
  Demux/1 -> Integrator_m/1
  dmEmb/1 -> Demux/1
  Demux/2 -> Integrator_E/1
  Demux/3 -> Integrator_mb/1
  Integrator_m/1 -> S-Function/1
  Integrator_E/1 -> S-Function/2
  Integrator_mb/1 -> S-Function/3
  dV/1 -> Integrator_V/1
  S-Function/1 -> p/1, Mux/1
  Mux/1 -> pTF/1
  S-Function/2 -> Mux/2
  Integrator_V/1 -> S-Function/4, v/1
  S-Function/3 -> Mux/3

== system EngineSystemSubmodel/Control Volume/ThdynCV_VarVolBus ==
  dm : Inport
  dE : Inport  Port=2
  dmb : Inport  Port=3
  dV : Inport  Port=4
  Bus Creator : BusCreator
  S-Function : S-Function  FunctionName=ThdynCVNV  Parameters=eng.fs,CV.m0,CV.E0,CV.mb0,CV.V0  SFunctionModules=GetThdynCombGasZach.c GetPTF.c  EnableBusSupport=off
  pTFV : Outport
  wires:
  dE/1 -> S-Function/2
  dm/1 -> S-Function/1
  dmb/1 -> S-Function/3
  dV/1 -> S-Function/4
  S-Function/2 -> Bus Creator/2  "T"
  S-Function/1 -> Bus Creator/1  "p"
  S-Function/3 -> Bus Creator/3  "F"
  S-Function/4 -> Bus Creator/4  "V"
  Bus Creator/1 -> pTFV/1

== system EngineSystemSubmodel/Emission/NOx ==
  pTFVBus : Inport
  phi : Inport  Port=2
  powCyl : Inport  Port=3
  Bus Selector : BusSelector  OutputSignals=p,T,F,Vb
  Constant : Constant  Value=1e-6
  Gain : Gain  Gain=30000
  Gain1 : Gain  Gain=1/3.6e6
  Gain2 : Gain  Gain=30
  Integrator : Integrator  ExternalReset=level
  Integrator1 : Integrator
  Integrator2 : Integrator
  Product : Product  Inputs=*/
  S-Function : S-Function  FunctionName=dNOxMol  Parameters=eng.fs, cyl.comb.T_L, cyl.comb.T_H, cyl.comb.FC, eng.xAir  EnableBusSupport=off
  S-Function1 : S-Function  FunctionName=resetCyc  Parameters=eng.nStroke  EnableBusSupport=off
  S-Function2 : S-Function  FunctionName=GetPerCycle  EnableBusSupport=off
  S-Function3 : S-Function  FunctionName=GetPerCycle  EnableBusSupport=off
  Sum : Sum  Inputs=|++
  NOxMolCyc : Outport
  sNOx : Outport  Port=2
  wCyc : Outport  Port=3
  NOxTotal : Outport  Port=4
  wires:
  Gain/1 -> sNOx/1
  Bus Selector/4 -> S-Function/4  "<Vb>"
  Bus Selector/3 -> S-Function/3  "<F>"
  Bus Selector/2 -> S-Function/2  "<T>"
  Bus Selector/1 -> S-Function/1  "<p>"
  S-Function/1 -> Integrator1/1, Integrator/1  "dNOxMol"
  Integrator/1 -> S-Function/5
  S-Function1/1 -> S-Function3/2, S-Function2/2, Integrator/2
  powCyl/1 -> Integrator2/1
  pTFVBus/1 -> Bus Selector/1
  Integrator2/1 -> S-Function2/1
  S-Function2/1 -> Sum/1  "wCyc"
  phi/1 -> S-Function1/1
  Integrator1/1 -> Gain2/1, S-Function3/1
  S-Function3/1 -> NOxMolCyc/1, Product/1  "NOxMolCyc"
  Product/1 -> Gain/1
  Sum/1 -> wCyc/1, Gain1/1
  Gain1/1 -> Product/2
  Constant/1 -> Sum/2
  Gain2/1 -> NOxTotal/1

== system EngineSystemSubmodel/EngineOperatingParameterCalculation/SFCCyc ==
  mqfCyc : Inport
  wCyc : Inport  Port=2
  resetCyc : Inport  Port=3
  S-Function : S-Function  FunctionName=SFCCyc  EnableBusSupport=off
  SFCCyc : Outport
  wires:
  mqfCyc/1 -> S-Function/1
  resetCyc/1 -> S-Function/3
  wCyc/1 -> S-Function/2
  S-Function/1 -> SFCCyc/1

== system EngineSystemSubmodel/EngineOperatingParameterCalculation/pCompCalc ==
  pCyl : Inport
  vCyl : Inport  Port=2
  tempWall : Inport  Port=3
  exhVVAOpen : Inport  Port=4
  S-Function2 : S-Function  FunctionName=pCompCalc  Parameters=vComp  EnableBusSupport=off  mask{vComp=vComp}
      mask prompts: vComp "Compression volume"
  Terminator : Terminator
  pComp : Outport
  wires:
  S-Function2/2 -> Terminator/1
  S-Function2/1 -> pComp/1
  exhVVAOpen/1 -> S-Function2/4
  tempWall/1 -> S-Function2/3
  vCyl/1 -> S-Function2/2
  pCyl/1 -> S-Function2/1

== system EngineSystemSubmodel/EngineOperatingParameterCalculation/pMaxFinder ==
  phi : Inport
  pCyl : Inport  Port=2
  Clock : Clock
      settings: Decimation=6
  S-Function : S-Function  FunctionName=pMaxFinder  EnableBusSupport=off
  pMax : Outport
  phiAtPMax : Outport  Port=2
  wires:
  S-Function/2 -> phiAtPMax/1
  S-Function/1 -> pMax/1
  pCyl/1 -> S-Function/3
  phi/1 -> S-Function/2
  Clock/1 -> S-Function/1

== system EngineSystemSubmodel/EngineOperatingParameterCalculation/resetCyc ==
  phi : Inport
  S-Function1 : S-Function  FunctionName=resetCyc  Parameters=eng.nStroke  EnableBusSupport=off
  reset : Outport
  wires:
  phi/1 -> S-Function1/1
  S-Function1/1 -> reset/1

== system EngineSystemSubmodel/EngineOperatingParameterCalculation/volEffCalc ==
  dmIntake : Inport
  pTFBus : Inport  Port=2
  omegaE : Inport  Port=3
  Bus Selector10 : BusSelector  OutputSignals=p,T
  Bus Selector9 : BusSelector  OutputSignals=R  OutputAsBus=on
  Gain2 : Gain  Gain=eng.cyl.dim.vD*eng.nCyl
  Gain3 : Gain  Gain=1/(eng.nStroke*pi)
  MovingAvg : Subsystem  mask{TdMA=5*1/(eng.RPMMax*0.5/60), y0=0}
      mask prompts: TdMA "Interval"; y0 "Initial Value"
  MovingAvg1 : Subsystem  mask{TdMA=5*1/(eng.RPMMax*0.5/60), y0=1e-5}
      mask prompts: TdMA "Interval"; y0 "Initial Value"
  Product : Product  Inputs=*//
  Product1 : Product
  Product2 : Product  Inputs=*/
  ThdynCombGasZach : EngineSystemSubmodel/ThermodynamicCalculation/ThdynCombGasZach
  volEff : Outport
  wires:
  Bus Selector10/2 -> Product/3  "<T>"
  Product1/1 -> MovingAvg1/1(in)
  Bus Selector9/1 -> Product/2
  pTFBus/1 -> Bus Selector10/1, ThdynCombGasZach/1
  ThdynCombGasZach/1 -> Bus Selector9/1
  Product/1 -> Gain2/1  "rhoAR"
  omegaE/1 -> Gain3/1
  MovingAvg/1(Out) -> Product2/1
  Gain2/1 -> Product1/1
  Bus Selector10/1 -> Product/1  "<p>"
  dmIntake/1 -> MovingAvg/1(in)
  Gain3/1 -> Product1/2  "cycPsec"
  Product2/1 -> volEff/1  "volEffCyl"
  MovingAvg1/1(Out) -> Product2/2

== system EngineSystemSubmodel/EngineOperatingParameterCalculation/workPerCycle ==
  powCyl : Inport
  phi : Inport  Port=2
  S-Function : S-Function  FunctionName=workPerCycle  Parameters=eng.nStroke  EnableBusSupport=off
  wCyc : Outport
  wires:
  S-Function/1 -> wCyc/1  "wCyc"
  powCyl/1 -> S-Function/1
  phi/1 -> S-Function/2

== system EngineSystemSubmodel/Flow Restriction/AirWaterCooler ==
  pTFu : Inport
  pTFd : Inport  Port=2
  TCW : Inport  Port=3
  Demux : Demux  Outputs=3
  Demux1 : Demux  Outputs=3
  Mux : Mux  Inputs=3
  Mux1 : Mux  Inputs=3
  S-Function : S-Function  FunctionName=AirWaterCoolerPTF  Parameters=eng.fs,cAC.Cd,cAC.areaAirPath,cAC.dmCW,cAC.coeffTCWK,cAC.CpCW,cAC.dCWPipe  SFunctionModules='GetAirDensity GetAirThermalConduct GetAirViscosity GetCompCombGas_rtwutil GetHTCoeffHTX GetIdealNozzleFlow GetThdynCombGasZach rt_nonfinite rtGetInf rtGetNaN'  EnableBusSupport=off
  dmEmbu : Outport
  dmEmbd : Outport  Port=2
  wires:
  S-Function/6 -> Mux1/3
  S-Function/5 -> Mux1/2
  S-Function/4 -> Mux1/1
  S-Function/3 -> Mux/3
  S-Function/2 -> Mux/2
  S-Function/1 -> Mux/1
  Demux/1 -> S-Function/1
  Demux/3 -> S-Function/3
  Demux/2 -> S-Function/2
  Demux1/3 -> S-Function/6
  Demux1/1 -> S-Function/4
  Demux1/2 -> S-Function/5
  pTFd/1 -> Demux1/1
  pTFu/1 -> Demux/1
  Mux/1 -> dmEmbu/1
  Mux1/1 -> dmEmbd/1
  TCW/1 -> S-Function/7

== system EngineSystemSubmodel/Flow Restriction/AirWaterCoolerBus ==
  pTFu : Inport
  pTFd : Inport  Port=2
  TCW : Inport  Port=3
  Bus Creator : BusCreator  Inputs=3
  Bus Creator1 : BusCreator  Inputs=3
  Bus Selector : BusSelector  OutputSignals=p,T,F
  Bus Selector1 : BusSelector  OutputSignals=p,T,F
  S-Function : S-Function  FunctionName=AirWaterCoolerPTF  Parameters=eng.fs,eng.cAC.Cd,eng.cAC.areaAirPath,eng.cAC.dmCW,eng.cAC.coeffTCWK,eng.cAC.CpCW,eng.cAC.dCWPipe  SFunctionModules='GetAirDensity GetAirThermalConduct GetAirViscosity GetCompCombGas_rtwutil GetHTCoeffHTX GetIdealNozzleFlow GetThdynCombGasZach rt_nonfinite rtGetInf rtGetNaN'  EnableBusSupport=off
  dmEmbu : Outport
  dmEmbd : Outport  Port=2
  wires:
  TCW/1 -> S-Function/7
  S-Function/1 -> Bus Creator/1  "dmu"
  S-Function/2 -> Bus Creator/2  "dEu"
  S-Function/3 -> Bus Creator/3  "dmbu"
  Bus Creator/1 -> dmEmbu/1
  S-Function/5 -> Bus Creator1/2  "dEd"
  S-Function/6 -> Bus Creator1/3  "dmbd"
  S-Function/4 -> Bus Creator1/1  "dmd"
  Bus Creator1/1 -> dmEmbd/1
  pTFu/1 -> Bus Selector/1
  pTFd/1 -> Bus Selector1/1
  Bus Selector/1 -> S-Function/1  "<p>"
  Bus Selector/2 -> S-Function/2  "<T>"
  Bus Selector/3 -> S-Function/3  "<F>"
  Bus Selector1/2 -> S-Function/5  "<T>"
  Bus Selector1/1 -> S-Function/4  "<p>"
  Bus Selector1/3 -> S-Function/6  "<F>"

== system EngineSystemSubmodel/Flow Restriction/Compressor ==
  pTF_u : Inport
  pTF_d : Inport  Port=2
  omegat : Inport  Port=3
  Demux : Demux  Outputs=3
  Demux1 : Demux  Outputs=3
  Mux : Mux  Inputs=3
  Mux1 : Mux  Inputs=3
  S-Function : S-Function  FunctionName=compressor_calc_PTF  Parameters=eng.fs,comp.flowMap,comp.effMap,comp.prRep,comp.n298Rep,int32(comp.npr),int32(comp.nsp)  SFunctionModules=GetThdynCombGasZach.c  EnableBusSupport=off
  dmEmb_u : Outport
  dmEmb_d : Outport  Port=2
  Tqt : Outport  Port=3
  eta_c : Outport  Port=4
  wires:
  Demux/1 -> S-Function/1
  Demux/3 -> S-Function/3
  Demux/2 -> S-Function/2
  Demux1/2 -> S-Function/5
  Demux1/3 -> S-Function/6
  Demux1/1 -> S-Function/4
  pTF_d/1 -> Demux1/1
  omegat/1 -> S-Function/7
  pTF_u/1 -> Demux/1
  S-Function/5 -> Mux1/2
  S-Function/4 -> Mux1/1
  S-Function/6 -> Mux1/3
  S-Function/1 -> Mux/1
  S-Function/2 -> Mux/2
  S-Function/3 -> Mux/3
  Mux/1 -> dmEmb_u/1
  Mux1/1 -> dmEmb_d/1
  S-Function/7 -> Tqt/1
  S-Function/8 -> eta_c/1

== system EngineSystemSubmodel/Flow Restriction/CompressorBus ==
  pTF_u : Inport
  pTF_d : Inport  Port=2
  omegat : Inport  Port=3
  Bus Creator : BusCreator  Inputs=3
  Bus Creator1 : BusCreator  Inputs=3
  Bus Selector : BusSelector  OutputSignals=p,T,F
  Bus Selector1 : BusSelector  OutputSignals=p,T,F
  S-Function : S-Function  FunctionName=compressor_calc_PTF  Parameters=eng.fs,turbo.comp.flowMap,turbo.comp.effMap,turbo.comp.prRep,turbo.comp.n288Rep,int32(turbo.comp.npr),int32(turbo.comp.nsp)  SFunctionModules=GetThdynCombGasZach.c  EnableBusSupport=off
  dmEmb_u : Outport
  dmEmb_d : Outport  Port=2
  Tqt : Outport  Port=3
  eta_c : Outport  Port=4
  wires:
  pTF_d/1 -> Bus Selector1/1
  pTF_u/1 -> Bus Selector/1
  Bus Selector/2 -> S-Function/2  "<T>"
  Bus Selector/3 -> S-Function/3  "<F>"
  Bus Selector/1 -> S-Function/1  "<p>"
  Bus Selector1/2 -> S-Function/5  "<T>"
  Bus Selector1/3 -> S-Function/6  "<F>"
  Bus Selector1/1 -> S-Function/4  "<p>"
  omegat/1 -> S-Function/7
  S-Function/2 -> Bus Creator/2  "dEu"
  S-Function/1 -> Bus Creator/1  "dmu"
  S-Function/3 -> Bus Creator/3  "dmbu"
  S-Function/5 -> Bus Creator1/2  "dEd"
  S-Function/4 -> Bus Creator1/1  "dmd"
  S-Function/6 -> Bus Creator1/3  "dmbd"
  S-Function/7 -> Tqt/1
  S-Function/8 -> eta_c/1
  Bus Creator/1 -> dmEmb_u/1
  Bus Creator1/1 -> dmEmb_d/1

== system EngineSystemSubmodel/Flow Restriction/CompressorFullMap ==
  pTFu : Inport
  pTFd : Inport  Port=2
  omegaT : Inport  Port=3
  Bus Creator2 : BusCreator  Inputs=3
  Bus Creator3 : BusCreator  Inputs=3
  Bus Selector : BusSelector  OutputSignals=p,T,F
  Bus Selector1 : BusSelector  OutputSignals=p,T,F
  S-Function : S-Function  FunctionName=compressor_calc_PTFV1  Parameters=eng.fs,comp.flowMap,comp.effMap,comp.prRep,comp.n298Rep,int32(comp.npr),int32(comp.nsp),int32(comp.nflow),comp.mDotRep  EnableBusSupport=off
  dmEmbu : Outport
  dmEmbd : Outport  Port=2
  tqC : Outport  Port=3
  etaComp : Outport  Port=4
  Td_calc : Outport  Port=5
  wires:
  S-Function/7 -> tqC/1  "tqT"
  Bus Selector/1 -> S-Function/1  "<p>"
  S-Function/5 -> Bus Creator3/2  "dEd"
  omegaT/1 -> S-Function/7
  pTFu/1 -> Bus Selector/1
  pTFd/1 -> Bus Selector1/1
  Bus Selector1/2 -> S-Function/5  "<T>"
  S-Function/2 -> Bus Creator2/2  "dEu"
  Bus Creator3/1 -> dmEmbd/1
  Bus Selector1/1 -> S-Function/4  "<p>"
  Bus Selector/3 -> S-Function/3  "<F>"
  Bus Selector/2 -> S-Function/2  "<T>"
  S-Function/6 -> Bus Creator3/3  "dmbd"
  S-Function/1 -> Bus Creator2/1  "dmu"
  Bus Selector1/3 -> S-Function/6  "<F>"
  S-Function/3 -> Bus Creator2/3  "dmbu"
  S-Function/4 -> Bus Creator3/1  "dmd"
  S-Function/8 -> etaComp/1  "etaComp"
  Bus Creator2/1 -> dmEmbu/1
  S-Function/9 -> Td_calc/1

== system EngineSystemSubmodel/Flow Restriction/IdealNozzle ==
  A_eff : Inport
  pTF_u : Inport  Port=2
  pTF_d : Inport  Port=3
  Demux : Demux  Outputs=3
  Demux1 : Demux  Outputs=3
  Mux : Mux  Inputs=3
  Mux1 : Mux  Inputs=3
  S-Function : S-Function  FunctionName=IdealNozzlePTF  Parameters=eng.fs  SFunctionModules='GetIdealNozzleFlw GetThdynCombGasZach GetCompCombGas_rtutil'  EnableBusSupport=off
  dmEmb_u : Outport
  dmEmb_d : Outport  Port=2
  wires:
  A_eff/1 -> S-Function/1
  pTF_u/1 -> Demux/1
  Demux/1 -> S-Function/2
  Demux/2 -> S-Function/3
  Demux/3 -> S-Function/4
  Demux1/1 -> S-Function/5
  Demux1/2 -> S-Function/6
  Demux1/3 -> S-Function/7
  pTF_d/1 -> Demux1/1
  S-Function/1 -> Mux/1
  S-Function/2 -> Mux/2
  S-Function/3 -> Mux/3
  S-Function/4 -> Mux1/1
  S-Function/5 -> Mux1/2
  S-Function/6 -> Mux1/3
  Mux/1 -> dmEmb_u/1
  Mux1/1 -> dmEmb_d/1

== system EngineSystemSubmodel/Flow Restriction/IdealNozzleBus ==
  A_eff : Inport
  pTF_u : Inport  Port=2
  pTF_d : Inport  Port=3
  Bus Creator : BusCreator  Inputs=3
  Bus Creator1 : BusCreator  Inputs=3
  Bus Selector : BusSelector  OutputSignals=p,T,F
  Bus Selector1 : BusSelector  OutputSignals=p,T,F
  S-Function : S-Function  FunctionName=IdealNozzlePTF  Parameters=eng.fs  SFunctionModules='GetIdealNozzleFlw GetThdynCombGasZach GetCompCombGas_rtutil'  EnableBusSupport=off
  dmEmb_u : Outport
  dmEmb_d : Outport  Port=2
  wires:
  A_eff/1 -> S-Function/1
  pTF_u/1 -> Bus Selector/1
  Bus Selector/1 -> S-Function/2  "<p>"
  Bus Selector/2 -> S-Function/3  "<T>"
  Bus Selector/3 -> S-Function/4  "<F>"
  Bus Selector1/1 -> S-Function/5  "<p>"
  Bus Selector1/2 -> S-Function/6  "<T>"
  Bus Selector1/3 -> S-Function/7  "<F>"
  pTF_d/1 -> Bus Selector1/1
  S-Function/1 -> Bus Creator/1  "dmu"
  S-Function/2 -> Bus Creator/2  "dEu"
  S-Function/3 -> Bus Creator/3  "dmbu"
  S-Function/4 -> Bus Creator1/1  "dmd"
  S-Function/5 -> Bus Creator1/2  "dEd"
  S-Function/6 -> Bus Creator1/3  "dmbd"
  Bus Creator/1 -> dmEmb_u/1
  Bus Creator1/1 -> dmEmb_d/1

== system EngineSystemSubmodel/Flow Restriction/Turbine ==
  pTF_u : Inport
  pTF_d : Inport  Port=2
  omegat : Inport  Port=3
  Demux : Demux  Outputs=3
  Demux1 : Demux  Outputs=3
  Mux : Mux  Inputs=3
  Mux1 : Mux  Inputs=3
  S-Function : S-Function  FunctionName=turbine_calc_PTF  Parameters=eng.fs,turb.flowCoeff,turb.effCoeff  SFunctionModules=GetThdynCombGasZach.c  EnableBusSupport=off
  dmEmb_u : Outport
  dmEmb_d : Outport  Port=2
  Tqt : Outport  Port=3
  Td_calc : Outport  Port=4
  effTurb : Outport  Port=5
  wires:
  Demux/1 -> S-Function/1
  Demux/3 -> S-Function/3
  Demux/2 -> S-Function/2
  Demux1/2 -> S-Function/5
  Demux1/3 -> S-Function/6
  Demux1/1 -> S-Function/4
  pTF_d/1 -> Demux1/1
  omegat/1 -> S-Function/7
  pTF_u/1 -> Demux/1
  S-Function/8 -> Td_calc/1
  S-Function/5 -> Mux1/2
  S-Function/4 -> Mux1/1
  S-Function/6 -> Mux1/3
  S-Function/1 -> Mux/1
  S-Function/2 -> Mux/2
  S-Function/3 -> Mux/3
  Mux/1 -> dmEmb_u/1
  Mux1/1 -> dmEmb_d/1
  S-Function/7 -> Tqt/1
  S-Function/9 -> effTurb/1
